simulink model "CurrentPI"  (R2020a)
settings: Solver=FixedStepAuto  StartTime=0.0  StopTime=10.0  FixedStep=1e-05  RelTol=1e-3
undefined symbols (not defined in the file or in its folder): Fsw
settings Model: DataDictionary=PCS_Simulation_EnviromentDD.sldd  Creator=ykamatan  LastModifiedBy=ykamatan
settings DataIOCC: SaveOutput=off  SaveTime=off
settings OptimizationCC: DefaultParameterBehavior=Inlined  EnhancedBackFolding=on  PassReuseOutputArgsAs=Individual arguments  ZeroExternalMemoryAtStartup=off  ZeroInternalMemoryAtStartup=off  OptimizeBlockOrder=speed  DifferentSizesBufferReuse=on  OptimizationCustomize=off  EfficientTunableParamExpr=on
settings DebuggingCC: ParameterTunabilityLossMsg=error
settings SFSimCC: MATLABDynamicMemAlloc=off
settings RTWCC: SystemTargetFile=ert.tlc  TemplateMakefile=ert_default_tmf
settings CodeAppCC: ForceParamTrailComments=on  IgnoreCustomStorageClasses=off  OperatorAnnotations=on  SimulinkDataObjDesc=on  SFDataObjDesc=on  InsertBlockDesc=on
settings ERTTargetCC: TargetLangStandard=C99 (ISO)  GenerateSampleERTMain=on  InlinedParameterPlacement=NonHierarchical  ERTCustomFileTemplate=example_file_process.tlc

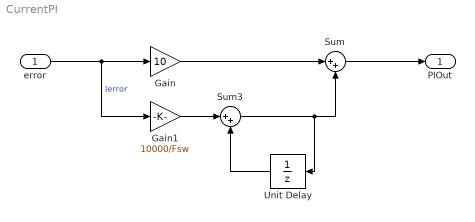
== system CurrentPI ==
  error : Inport  OutDataTypeStr=double  PortDimensions=1  SampleTime=[1.0000000000000001e-05,0]
  Gain : Gain  Gain=10
  Gain1 : Gain  Gain=10000/Fsw
  Sum : Sum  Inputs=|++
  Sum3 : Sum  Inputs=|++
  Unit Delay : UnitDelay  SampleTime=1/Fsw  HasFrameUpgradeWarning=on
  PIOut : Outport  OutDataTypeStr=double  PortDimensions=1  SampleTime=[1.0000000000000001e-05,0]
  wires:
  Unit Delay/1 -> Sum3/2
  error/1 -> Gain/1, Gain1/1  "Ierror"
  Sum/1 -> PIOut/1
  Gain/1 -> Sum/1
  Gain1/1 -> Sum3/1
  Sum3/1 -> Sum/2, Unit Delay/1
